simulink model "simu"  (R2022b)
settings: Solver=VariableStepAuto  StartTime=0.0  StopTime=30  RelTol=1e-3
values from neighbouring files (symbols this model uses):
  c = 2    [matlab.mat]
  d = 4    [matlab.mat]
settings Model: NumberOfSteps=5  Creator=paola  LastModifiedBy=paola

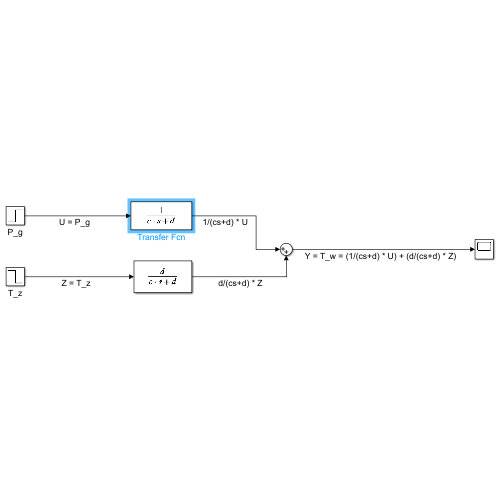
[thumbnail: Simulink's stored preview of the top-level diagram]
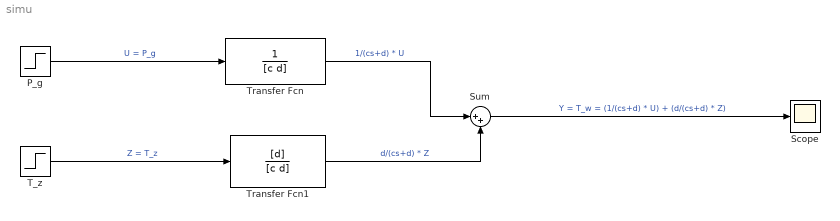
== system simu ==
  P_g : Step  After=0  SampleTime=0
  Scope : Scope
  Sum : Sum  Inputs=|++
  T_z : Step  Time=2  After=-2  SampleTime=0
  Transfer Fcn : TransferFcn  Denominator=[c d]
  Transfer Fcn1 : TransferFcn  Numerator=[d]  Denominator=[c d]
  wires:
  P_g/1 -> Transfer Fcn/1  "U = P_g"
  T_z/1 -> Transfer Fcn1/1  "Z = T_z"
  Sum/1 -> Scope/1  "Y = T_w = (1/(cs+d) * U) + (d/(cs+d) * Z)"
  Transfer Fcn/1 -> Sum/1  "1/(cs+d) * U"
  Transfer Fcn1/1 -> Sum/2  "d/(cs+d) * Z"
